simulink model "convert"  (R2022a)
settings: Solver=FixedStepAuto  StartTime=0.0  StopTime=1  FixedStep=Ts  RelTol=1e-3
model workspace (MAT data in the model file):
  B = 1
  Ts = Simulink.Parameter
  Ts.Value = 0.01
  Ts.DataType = 'auto'
  Ts.Complexity = 'real'
  Ts.Dimensions = [1 1]
  a = Simulink.Parameter
  a.Value = -1
  a.DataType = 'auto'
  a.Complexity = 'real'
  a.Dimensions = [1 1]
  d = Simulink.Parameter
  d.Value = 0.3
  d.DataType = 'auto'
  d.Complexity = 'real'
  d.Dimensions = [1 1]
  lamda = Simulink.Parameter
  lamda.Value = 0.37
  lamda.DataType = 'auto'
  lamda.Complexity = 'real'
  lamda.Dimensions = [1 1]
  w = Simulink.Parameter
  w.Value = 1.2
  w.DataType = 'auto'
  w.Complexity = 'real'
  w.Dimensions = [1 1]
settings Model: Creator=xzhao  LastModifiedBy=xzhao
settings OptimizationCC: DefaultParameterBehavior=Inlined  EnhancedBackFolding=on  PassReuseOutputArgsAs=Individual arguments  ZeroExternalMemoryAtStartup=off  ZeroInternalMemoryAtStartup=off  OptimizeBlockOrder=speed  DifferentSizesBufferReuse=on  OptimizationCustomize=off  EfficientTunableParamExpr=on
settings DebuggingCC: ParameterTunabilityLossMsg=error
settings HardwareCC: TargetBitPerPointer=64  TargetBitPerSizeT=64  TargetBitPerPtrDiffT=64  TargetLongLongMode=on  TargetIntDivRoundTo=Zero  TargetEndianess=LittleEndian  TargetWordSize=64  TargetHWDeviceType=MATLAB Host  ProdEqTarget=off
settings SFSimCC: MATLABDynamicMemAlloc=off
settings RTWCC: Description=Embedded Coder (host-based shared library target)  SystemTargetFile=ert_shrlib.tlc  TemplateMakefile=ert_default_tmf
settings CodeAppCC: ForceParamTrailComments=on  IgnoreCustomStorageClasses=off  OperatorAnnotations=on  SimulinkDataObjDesc=on  SFDataObjDesc=on  InsertBlockDesc=on
settings STFCustomTargetCC: TargetLangStandard=C99 (ISO)  MultiwordLength=256  GenerateSampleERTMain=on  ParMdlRefBuildCompliant=on  CompOptLevelCompliant=on  CombineOutputUpdateFcns=on  ERTCustomFileBanners=on  SupportContinuousTime=off  SupportNonInlinedSFcns=off  RemoveResetFunc=on  MATLABClassNameForMDSCustomization=Simulink.SoftwareTarget.ERTCustomization  ModelStepFunctionPrototypeControlCompliant=on  GRTInterface=off  UseToolchainInfoCompliant=on  SystemTargetFile=ert_shrlib.tlc
settings ERTTargetCC: TargetLangStandard=C99 (ISO)  GenerateSampleERTMain=on  ConcurrentExecutionCompliant=off  CPPClassGenCompliant=off  InlinedParameterPlacement=NonHierarchical  ERTCustomFileTemplate=example_file_process.tlc

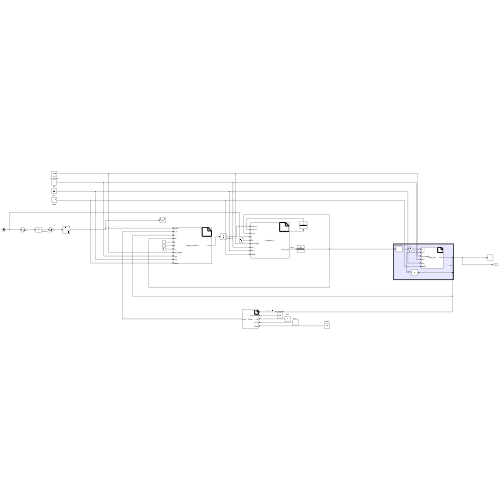
[thumbnail: Simulink's stored preview of the top-level diagram]
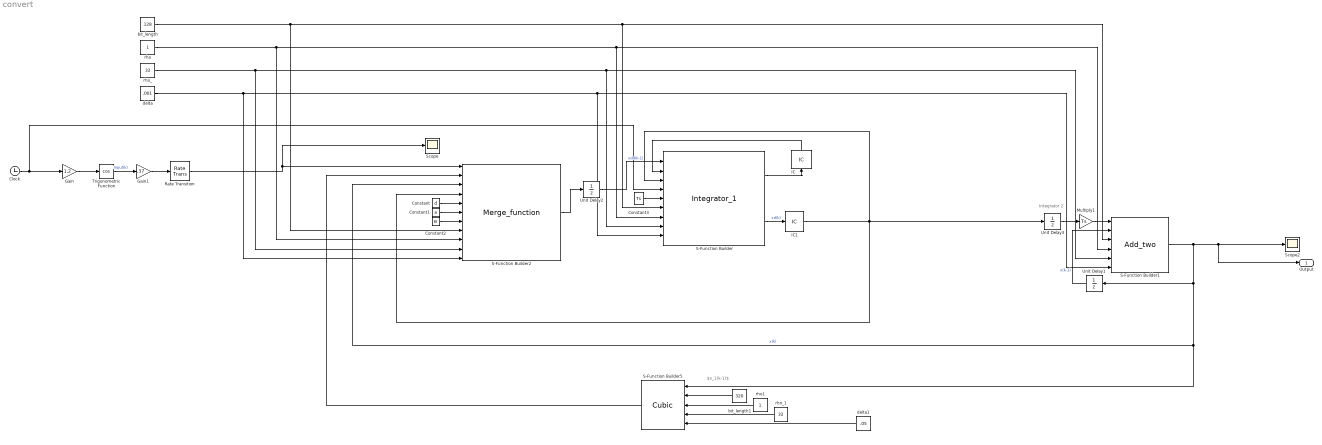
== system convert ==
  note: $x_1(k-1)$
  note: Integrator 2
  Clock : Clock
  Constant : Constant  Value=d
  Constant1 : Constant  Value=a
  Constant2 : Constant  Value=B
  Constant3 : Constant  Value=Ts
  Gain : Gain  Gain=1.2
  Gain1 : Gain  Gain=.37
  IC : InitialCondition  Value=0
  IC1 : InitialCondition  Value=0
  Multiply1 : Gain  Gain=Ts
  Rate Transition : RateTransition  OutPortSampleTime=Ts
  S-Function Builder : S-Function  FunctionName=Integrator_1  SFunctionModules=Integrator_1_wrapper  SFunctionDeploymentMode=off  EnableBusSupport=off  mask(S-Function Builder){}
      mask help: Simulink:masks:SFunctionBuilder_MD
      mask init:
      | val = [[.9  0.75 0.75 1 1 .9 .9 1]',[1 1 0.75 0.75 .9 .9 1 .9]'];try , sys = get_param(gcb,'SfunBuilderFcnName');if isempty(sys), sys = get_param(gcb,'FunctionName'); end,catch, sys = get_param(gcb,'FunctionName'); end
      settings: CopyFcn=set_param(gcbh,'LinkStatus','none')  OpenFcn=sfunctionwizard(gcbh)
      mask Display:
      | plot(val(:,1),val(:,2))
      | disp(sys)
      | port_label('input',1,'xdd_m1')
      | port_label('input',2,'xd_m1')
      | port_label('input',3,'xd_k')
      | port_label('input',4,'t')
      | port_label('input',5,'Ts')
      | port_label('input',6,'bit_length')
      | port_label('input',7,'rho')
      | port_label('input',8,'rho_')
      | port_label('input',9,'delta')
      | port_label('output',1,'xd_m1_out')
      | port_label('output',2,'xd_k_out')
  S-Function Builder1 : S-Function  FunctionName=Add_two  Parameters=1  SFunctionModules=Add_two_wrapper  SFunctionDeploymentMode=off  EnableBusSupport=off  mask(S-Function Builder){}
      mask help: Simulink:masks:SFunctionBuilder_MD
      mask init: same as convert/S-Function Builder
      settings: CopyFcn=set_param(gcbh,'LinkStatus','none')  OpenFcn=sfunctionwizard(gcbh)
      mask Display:
      | plot(val(:,1),val(:,2))
      | disp(sys)
      | port_label('input',1,'x_1')
      | port_label('input',2,'x_2')
      | port_label('input',3,'bit_length')
      | port_label('input',4,'rho')
      | port_label('input',5,'rho_')
      | port_label('input',6,'delta')
      | port_label('output',1,'sum')
  S-Function Builder2 : S-Function  FunctionName=Merge_function  SFunctionModules=Merge_function_wrapper  SFunctionDeploymentMode=off  EnableBusSupport=off  mask(S-Function Builder){}
      mask help: Simulink:masks:SFunctionBuilder_MD
      mask init: same as convert/S-Function Builder
      settings: CopyFcn=set_param(gcbh,'LinkStatus','none')  OpenFcn=sfunctionwizard(gcbh)
      mask Display:
      | plot(val(:,1),val(:,2))
      | disp(sys)
      | port_label('input',1,'input')
      | port_label('input',2,'x_3')
      | port_label('input',3,'x')
      | port_label('input',4,'xd')
      | port_label('input',5,'d')
      | port_label('input',6,'a')
      | port_label('input',7,'b')
      | port_label('input',8,'bit_length')
      | port_label('input',9,'rho')
      | port_label('input',10,'rho_')
      | port_label('input',11,'delta')
      | port_label('output',1,'sum')
  S-Function Builder5 : S-Function  FunctionName=Cubic  SFunctionModules=Cubic_wrapper  SFunctionDeploymentMode=off  EnableBusSupport=off  mask(S-Function Builder){}
      mask help: Simulink:masks:SFunctionBuilder_MD
      mask init: same as convert/S-Function Builder
      settings: CopyFcn=set_param(gcbh,'LinkStatus','none')  OpenFcn=sfunctionwizard(gcbh)
      mask Display:
      | plot(val(:,1),val(:,2))
      | disp(sys)
      | port_label('input',1,'x')
      | port_label('input',2,'bit_length')
      | port_label('input',3,'rho')
      | port_label('input',4,'rho_')
      | port_label('input',5,'delta')
      | port_label('output',1,'sum')
  Scope : Scope
  Scope2 : Scope
  Trigonometric Function : Trigonometry  Operator=cos
  Unit Delay1 : UnitDelay  InitialCondition=1  SampleTime=-1  HasFrameUpgradeWarning=on
  Unit Delay2 : UnitDelay  SampleTime=-1  HasFrameUpgradeWarning=on
  Unit Delay3 : UnitDelay  SampleTime=-1  HasFrameUpgradeWarning=on
  bit_length : Constant  Value=128
  bit_length1 : Constant  Value=320
  delta : Constant  Value=.001
  delta1 : Constant  Value=.05
  rho : Constant
  rho1 : Constant
  rho_ : Constant  Value=32
  rho_1 : Constant  Value=32
  Output : Outport
  wires:
  Trigonometric Function/1 -> Gain1/1  "input(k)"
  S-Function Builder/2 -> IC1/1  "xd(k)"
  Multiply1/1 -> S-Function Builder1/1
  S-Function Builder1/1 -> S-Function Builder2/3, S-Function Builder5/1, Unit Delay1/1, Output/1, Scope2/1  "x(k)"
  Unit Delay1/1 -> S-Function Builder1/2  "x(k-1)"
  Unit Delay3/1 -> Multiply1/1
  Clock/1 -> S-Function Builder/4, Gain/1
  Gain/1 -> Trigonometric Function/1
  Gain1/1 -> Rate Transition/1
  Rate Transition/1 -> S-Function Builder2/1, Scope/1
  rho/1 -> S-Function Builder2/9, S-Function Builder/7, S-Function Builder1/4
  rho_/1 -> S-Function Builder2/10, S-Function Builder/8, S-Function Builder1/5
  bit_length/1 -> S-Function Builder2/8, S-Function Builder1/3, S-Function Builder/6
  delta/1 -> S-Function Builder2/11, S-Function Builder1/6, S-Function Builder/9
  bit_length1/1 -> S-Function Builder5/2
  rho1/1 -> S-Function Builder5/3
  rho_1/1 -> S-Function Builder5/4
  delta1/1 -> S-Function Builder5/5
  Constant/1 -> S-Function Builder2/5
  Constant1/1 -> S-Function Builder2/6
  Constant2/1 -> S-Function Builder2/7
  S-Function Builder2/1 -> Unit Delay2/1
  S-Function Builder5/1 -> S-Function Builder2/2
  S-Function Builder/1 -> IC/1
  Unit Delay2/1 -> S-Function Builder/1  "xdd(k-1)"
  Constant3/1 -> S-Function Builder/5
  IC/1 -> S-Function Builder/2
  IC1/1 -> S-Function Builder2/4, S-Function Builder/3, Unit Delay3/1
